simulink model "Centre_tapped"  (R2024a)
settings: Solver=FixedStepAuto  StartTime=0.0  StopTime=0.1  RelTol=1e-3
libraries: spsThyristorLib x2, spsACVoltageSourceLib x1, spsCurrentMeasurementLib x1, spsGroundLib x1, spsLinearTransformerLib x1, spsSeriesRLCBranchLib x1, spsVoltageMeasurementLib x1, spspowerguiLib x1
settings Model: Creator=adity  LastModifiedBy=adity

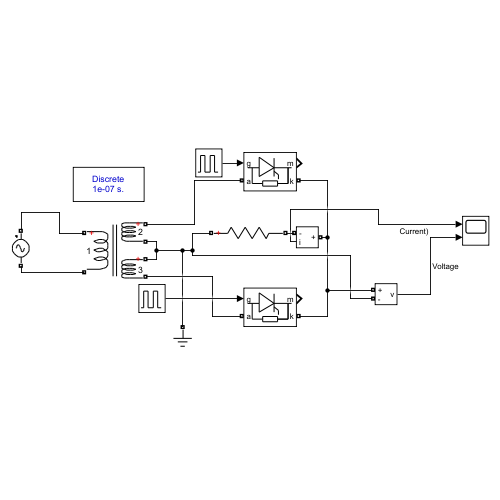
[thumbnail: Simulink's stored preview of the top-level diagram]
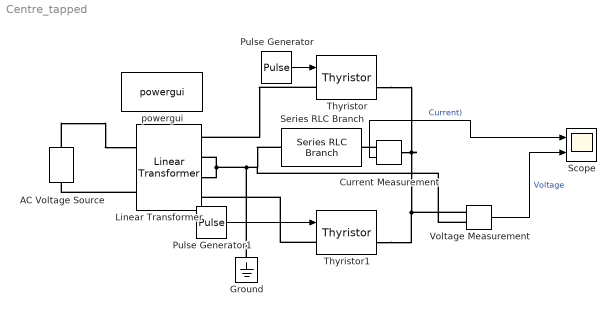
== system Centre_tapped ==
  AC Voltage Source : spsACVoltageSourceLib/AC Voltage Source  Amplitude=220  Phase=0  Frequency=50  SampleTime=0  Measurements=None  BusType=swing  Pref=10e3  Qref=0  Qmin=-inf  Qmax=+inf
  Current Measurement : spsCurrentMeasurementLib/Current Measurement  PhasorSimulation=off  OutputType=Complex  PSBequivalent=0
  Ground : spsGroundLib/Ground  LConnTagsString=a
  Linear Transformer : spsLinearTransformerLib/Linear Transformer  UNITS=SI  NominalPower=[1000 50]  winding1=[220 0.1 0]  winding2=[155 0.1 0]  ThreeWindings=on  winding3=[155 0.1 0]  RmLm=[500 500]  Measurements=None  DataType=on
  Pulse Generator : DiscretePulseGenerator  PulseType=Time based  Period=0.02  PulseWidth=5  PhaseDelay=0.00056
  Pulse Generator1 : DiscretePulseGenerator  PulseType=Time based  Period=0.02  PulseWidth=5  PhaseDelay=0.01056
  Scope : Scope  NumInputPorts=2
  Series RLC Branch : spsSeriesRLCBranchLib/Series RLC Branch  LConnTagsString=__new0  RConnTagsString=__new0  BranchType=R  Resistance=1  Inductance=1e-3  SetiL0=off  InitialCurrent=0  Capacitance=1e-6  Setx0=off  InitialVoltage=0  Measurements=None
  Thyristor : spsThyristorLib/Thyristor  Ron=0.001  Lon=0  Vf=0.8  IC=0  Rs=500  Cs=250e-9  Measurements=on
  Thyristor1 : spsThyristorLib/Thyristor  Ron=0.001  Lon=0  Vf=0.8  IC=0  Rs=500  Cs=250e-9  Measurements=on
  Voltage Measurement : spsVoltageMeasurementLib/Voltage Measurement  PhasorSimulation=off  OutputType=Complex  PSBequivalent=0
  powergui : spspowerguiLib/powergui  Priority=1  SimulationMode=Discrete  SampleTime=1e-7  frequency=60  Iterations=50  frequencyindice=50  Pbase=100e6  ErrMax=1e-4  UnitsV=kV  UnitsW=MW  buscounter=0  FunctionMessages=off  echomessages=off  EnableUseOfTLC=off  CurrentSourceSwitches=off  DisableSnubberDevices=off  DisableRonSwitches=off  DisableVfSwitches=off  DisplayEquations=off  AutomaticDiscreteSolvers=off  SolverType=Tustin/Backward Euler (TBE)  Interpol=off  ExternalGateDelay=off  methode=off  Ts=100  x0status=blocks  SPID=on  SwTol=0  HookPort=off  NonlinearTolerance=1e-4  nMaxIteration=100  ContinueOnMaxIteration=off  RestoreLinks=warning  ResistiveCurrentMeasurement=off  Frange=[0:2:500]  Ylog=off  Xlog=on  ShowGrid=off  save=off  variable=ZData  structure=0  ZoomFFT=off  StartTime=0.0  cycles=1  DisplayStyle=1  fundamental=60  FreqAxis=off  MaxFrequency=1000  frequencyindicesteady=1  RmsSteady=1  display=off
  wires:
  Pulse Generator/1 -> Thyristor/1
  Pulse Generator1/1 -> Thyristor1/1
  Voltage Measurement/1 -> Scope/2  "Voltage"
  Current Measurement/1 -> Scope/1  "Current)"
  connections:
  Thyristor/LConn1 -- Linear Transformer/RConn1
  Thyristor1/LConn1 -- Linear Transformer/RConn4
  Linear Transformer/RConn3 -- Voltage Measurement/LConn2 -- Series RLC Branch/LConn1 -- Ground/LConn1 -- Linear Transformer/RConn2
  AC Voltage Source/RConn1 -- Linear Transformer/LConn1
  Linear Transformer/LConn2 -- AC Voltage Source/LConn1
  Thyristor/RConn1 -- Current Measurement/LConn1 -- Thyristor1/RConn1 -- Voltage Measurement/LConn1
  Current Measurement/RConn1 -- Series RLC Branch/RConn1
